simulink model "circular_discreto"  (R2017a)
settings: Solver=VariableStepAuto  StartTime=0.0  StopTime=15  RelTol=1e-3
values from neighbouring files (symbols this model uses):
  C = [1 0 0]    [principal.m]
  Gd = sysd.A    [principal.m]
  Hd = sysd.B    [principal.m]
undefined symbols (not defined in the file or in its folder): DiscIntNeverNeededParam, Discrete, K_lqrd, Time
libraries: simulink x3, ctrlSharedLib x2
settings Model: Creator=dscat  LastModifiedBy=dscat

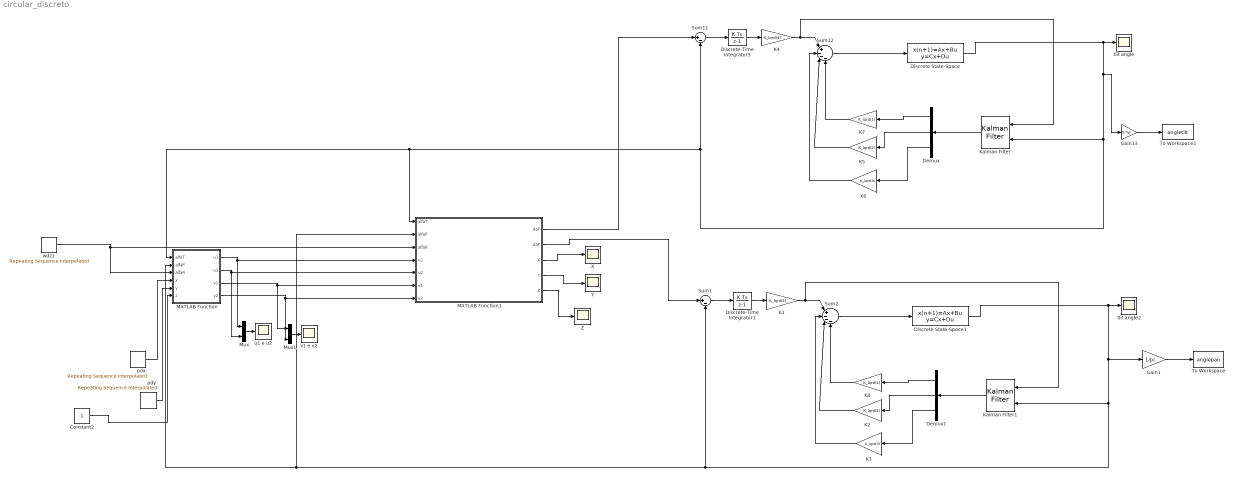
== system circular_discreto ==
  Constant2 : Constant
  Demux : Demux  Outputs=3
  Demux1 : Demux  Outputs=3
  Discrete State-Space : DiscreteStateSpace  A=Gd  B=Hd  C=C  D=0  SampleTime=0.05
  Discrete State-Space1 : DiscreteStateSpace  A=Gd  B=Hd  C=C  D=0  SampleTime=0.05
  Discrete-Time Integrator1 : DiscreteIntegrator  InitialConditionSetting=State (most efficient)  SampleTime=0.05  ICPrevOutput=DiscIntNeverNeededParam  ICPrevScaledInput=DiscIntNeverNeededParam
  Discrete-Time Integrator3 : DiscreteIntegrator  InitialConditionSetting=State (most efficient)  SampleTime=0.05  ICPrevOutput=DiscIntNeverNeededParam  ICPrevScaledInput=DiscIntNeverNeededParam
  Gain1 : Gain  Gain=1/pi
  Gain13 : Gain  Gain=0.7/pi
  K1 : Gain  Gain=-K_lqrd(4)
  K2 : Gain  Gain=K_lqrd(2)
  K3 : Gain  Gain=K_lqrd(3)
  K4 : Gain  Gain=-K_lqrd(4)
  K5 : Gain  Gain=K_lqrd(2)
  K6 : Gain  Gain=K_lqrd(3)
  K7 : Gain  Gain=K_lqrd(1)
  K8 : Gain  Gain=K_lqrd(1)
  Kalman Filter : ctrlSharedLib/Kalman Filter  TimeDomain=Discrete-Time  UseCurrentEstimator=on  ModelSource=LTI State-Space Variable  ModelSourceVariable=sysd  A=0.95  B=1  C=1  D=0  NumberOfStates=1  NumberOfInputs=1  NumberOfOutputs=1  InitialEstimateSource=Dialog  X0=0  P0=10  UseK=off  UseGH=off  NumberOfProcessNoiseInputs=1  G=1  TimeInvariantG=on  H=0  TimeInvariantH=on  Q=0.1  TimeInvariantQ=on  R=0.5  TimeInvariantR=on  N=0  TimeInvariantN=on  AddInputPort=on  AddEnablePort=off  OutputEstimatedY=off  OutputP=off  Ts=-1
  Kalman Filter1 : ctrlSharedLib/Kalman Filter  TimeDomain=Discrete-Time  UseCurrentEstimator=on  ModelSource=LTI State-Space Variable  ModelSourceVariable=sysd  A=0.95  B=1  C=1  D=0  NumberOfStates=1  NumberOfInputs=1  NumberOfOutputs=1  InitialEstimateSource=Dialog  X0=0  P0=10  UseK=off  UseGH=off  NumberOfProcessNoiseInputs=1  G=1  TimeInvariantG=on  H=0  TimeInvariantH=on  Q=0.1  TimeInvariantQ=on  R=0.5  TimeInvariantR=on  N=0  TimeInvariantN=on  AddInputPort=on  AddEnablePort=off  OutputEstimatedY=off  OutputP=off  Ts=-1
  MATLAB Function : MATLAB Function  TreatAsAtomicUnit=on
  MATLAB Function1 : MATLAB Function  TreatAsAtomicUnit=on
  Mux : Mux  Inputs=2
  Mux1 : Mux  Inputs=2
  Sum1 : Sum  Inputs=|+-
  Sum11 : Sum  Inputs=|+-
  Sum12 : Sum  Inputs=|+---
  Sum2 : Sum  Inputs=|+---
  To Workspace : ToWorkspace  VariableName=anglepan  SampleTime=-1
      settings: MaxDataPoints=1
  To Workspace1 : ToWorkspace  VariableName=angletilt  SampleTime=0.05
      settings: MaxDataPoints=1
  X : Scope
  Y : Scope
  Z : Scope
  pdx : simulink/Sources/Repeating Sequence Interpolated  OutValues=pdx  TimeValues=t  LookUpMeth=Interpolation-Use End Values  tsamp=0.01  OutMin=[]  OutMax=[]  OutDataTypeStr=double  OutputDataTypeScalingMode=double  OutDataType=fixdt(0,8)  OutScaling=2^-10
  pdy : simulink/Sources/Repeating Sequence Interpolated  OutValues=pdy  TimeValues=t  LookUpMeth=Interpolation-Use End Values  tsamp=0.01  OutMin=[]  OutMax=[]  OutDataTypeStr=double  OutputDataTypeScalingMode=double  OutDataType=fixdt(0,8)  OutScaling=2^-10
  tlit angle : Scope
  tlit angle2 : Scope
  u1 e u2 : Scope
  v1 e v2 : Scope
  wdz1 : simulink/Sources/Repeating Sequence Interpolated  OutValues=wdz  TimeValues=t  LookUpMeth=Interpolation-Use End Values  tsamp=0.01  OutMin=[]  OutMax=[]  OutDataTypeStr=double  OutputDataTypeScalingMode=double  OutDataType=fixdt(0,8)  OutScaling=2^-10
  wires:
  MATLAB Function/2(u2) -> MATLAB Function1/5(u2), Mux/2
  Constant2/1 -> MATLAB Function/6(z)
  MATLAB Function1/5(Z) -> Z/1
  MATLAB Function/4(v2) -> MATLAB Function1/7(v2), Mux1/2
  MATLAB Function/1(u1) -> MATLAB Function1/4(u1), Mux/1
  pdx/1 -> MATLAB Function/4(x)
  pdy/1 -> MATLAB Function/5(y)
  MATLAB Function1/4(Y) -> Y/1
  Mux/1 -> u1 e u2/1
  wdz1/1 -> MATLAB Function1/3(alfaR), MATLAB Function/3(alfaR)
  Mux1/1 -> v1 e v2/1
  MATLAB Function/3(v1) -> MATLAB Function1/6(v1), Mux1/1
  MATLAB Function1/3(X) -> X/1
  K5/1 -> Sum12/3
  Discrete-Time Integrator3/1 -> K4/1
  Sum11/1 -> Discrete-Time Integrator3/1
  Demux/3 -> K6/1
  Discrete State-Space/1 -> Gain13/1, MATLAB Function/1(alfaT), MATLAB Function1/1(alfaT), Sum11/2, Kalman Filter/2, tlit angle/1
  K4/1 -> Kalman Filter/1, Sum12/1
  MATLAB Function1/1(daT) -> Sum11/1
  Demux/1 -> K7/1
  K6/1 -> Sum12/2
  Demux/2 -> K5/1
  Kalman Filter/1 -> Demux/1
  Sum12/1 -> Discrete State-Space/1
  K7/1 -> Sum12/4
  Gain13/1 -> To Workspace1/1
  Demux1/1 -> K8/1
  K3/1 -> Sum2/2
  MATLAB Function1/2(daP) -> Sum1/1
  K1/1 -> Kalman Filter1/1, Sum2/1
  Kalman Filter1/1 -> Demux1/1
  Sum2/1 -> Discrete State-Space1/1
  K8/1 -> Sum2/4
  K2/1 -> Sum2/3
  Demux1/3 -> K3/1
  Gain1/1 -> To Workspace/1
  Sum1/1 -> Discrete-Time Integrator1/1
  Discrete State-Space1/1 -> MATLAB Function/2(alfaP), MATLAB Function1/2(alfaP), Sum1/2, Kalman Filter1/2, Gain1/1, tlit angle2/1
  Discrete-Time Integrator1/1 -> K1/1
  Demux1/2 -> K2/1

== matlab function circular_discreto/MATLAB Function1 ==
  data: alfaT input; daT output; alfaP input; alfaR input; u1 input; u2 input; v1 input; v2 input; daP output; X output; Y output; Z output
function [daT, daP, X,Y,Z  ] = image2real( alfaT,alfaP,alfaR, u1,u2,v1,v2)
% daT -> Delta Alfa Tilt
% daP -> Delta Alfa Pan
% AlfaR -> Lido dos encoders


l = 0.15; %Tamanho do alvo (m) 
f = 664;

X = (l*(f*cos(alfaP-alfaR) - u2*sin(alfaP-alfaR))*(- cos(alfaP-alfaR)*sin(alfaP-alfaR)*f^2 + (u1 - cos(alfaP-alfaR)^2*(u1 + u2))*f + u1*u2*cos(alfaP-alfaR)*sin(alfaP-alfaR)))/(f*(u2*cos(alfaP-alfaR) + f*sin(alfaP-alfaR))*(u1 - u2));

%X = (l*(f*cos(alfaT) - v2*sin(alfaT))*(- cos(alfaT)*sin(alfaT)*f^2 + (v1 - cos(alfaT)^2*(v1 + v2))*f + v1*v2*cos(alfaT)*sin(alfaT)))/(f*(f*sin(alfaT) + v2*cos(alfaT))*(v1 - v2));

Y = -(l*(2*cos(alfaP-alfaR)*sin(alfaP-alfaR)*f^2 + (u1 + u2)*(2*cos(alfaP-alfaR)^2 - 1)*f - 2*u1*u2*cos(alfaP-alfaR)*sin(alfaP-alfaR)))/(2*f*(u1 - u2));

Z  = -(l*(2*cos(alfaT)*sin(alfaT)*f^2 + (v1 + v2)*(2*cos(alfaT)^2 - 1)*f - 2*v1*v2*cos(alfaT)*sin(alfaT)))/(2*f*(v1 - v2));
 
daP = double(atan(Y/X)+alfaR);
%daT = double(atan(Z/(sqrt((X)^2+(Y)^2))));
daT = double(atan(Z/X));

end

== matlab function circular_discreto/MATLAB Function ==
  data: alfaT input; u1 output; alfaP input; alfaR input; x input; y input; z input; u2 output; v1 output; v2 output
function [u1, u2, v1, v2] = real2image(alfaT,alfaP,alfaR,x,y,z)
L = 0.15;
f = 664;
u1 = f*(-sin(alfaP-alfaR)*(-x)+cos(alfaP-alfaR)*((L/2)-y))/((cos(alfaP-alfaR)*(-x)+sin(alfaP-alfaR)*((L/2)-y)));
u2 = f*(-sin(alfaP-alfaR)*(-x)+cos(alfaP-alfaR)*((-L/2)-y))/((cos(alfaP-alfaR)*(-x)+sin(alfaP-alfaR)*((-L/2)-y)));
v1 = f*(-sin(alfaT)*(-x)+cos(alfaT)*((L/2)-z))/((cos(alfaT)*(-x)+sin(alfaT)*((L/2)-z)));
v2 = f*(-sin(alfaT)*(-x)+cos(alfaT)*((-L/2)-z))/((cos(alfaT)*(-x)+sin(alfaT)*((-L/2)-z)));

end
